simulink library "MicDiagBtc"  (R2022b)
settings: Solver=VariableStepAuto  StartTime=0.0  StopTime=10.0  RelTol=1e-3
libraries: RTC x2, FeaturePath x1, HandyTextFile x1, simulink x1
settings Model: Creator=yp1048186  LastModifiedBy=kl13806
settings SolverCC: AlgebraicLoopSolver=TrustRegion
settings DebuggingCC: UnconnectedInputMsg=warning  UnconnectedOutputMsg=warning  UnconnectedLineMsg=warning  SFMachineParentedDataDiag=warning
settings ModelReferenceCC: EnableRefExpFcnMdlSchedulingChecks=on
settings RTWCC: DLArmComputeVersion=19.05

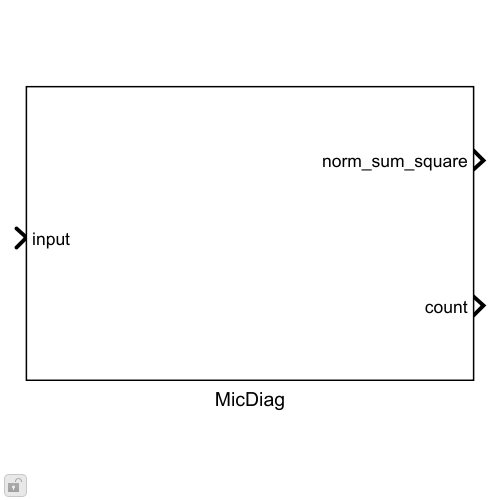
[thumbnail: Simulink's stored preview of the top-level diagram]
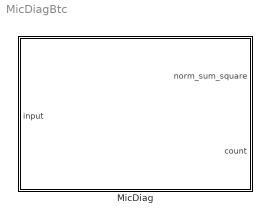
== system MicDiagBtc ==
  MicDiag : Subsystem  mask(Blocklib MicDiag){Config=[], FeatureName=MicDiag}
      mask prompts: Config "MicDiagConfig"; FeatureName "Feature path name:"
      mask help: MicDiag accumulates the sum of squares for multiple channels individually
      mask init:
      | blkh=gcbh;
      | Config=BTConfig.Assert(blkh,Config);
      | 
      | Config.Validate();
      | BTConfig.InitSetFeatureIfPresent(blkh,'FeatureName');
      mask Callback Config: BTConfig.CallbackHideIfPresent(gcbh,{'FeatureName'});
      mask TypeOptions FeatureName: FeaturePath/FeatureName

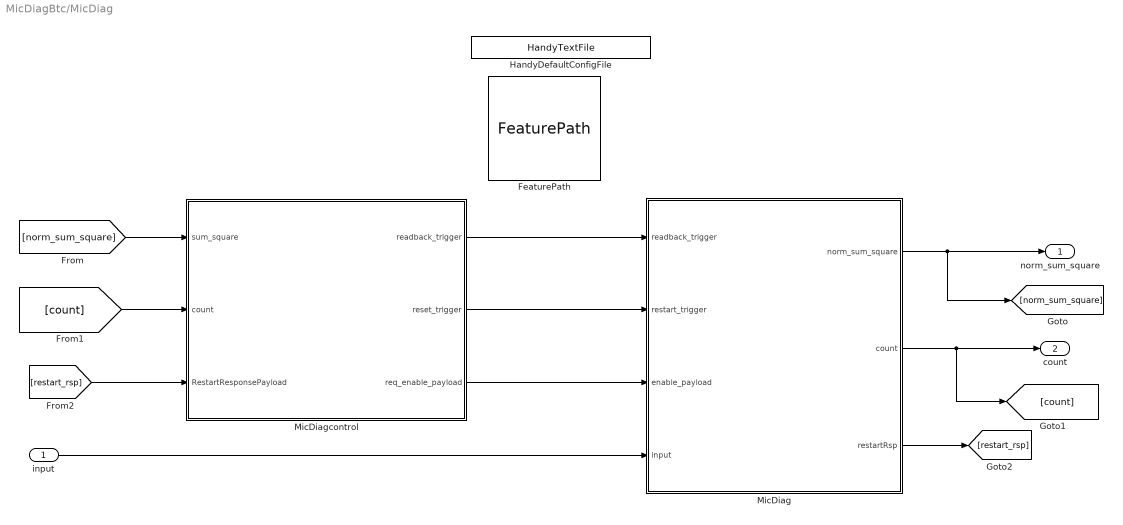
== system MicDiagBtc/MicDiag ==
  input : Inport
  FeaturePath : FeaturePath/FeaturePath  FeatureName=MicDiag  IsGroup=off  GroupNumber=-1  IsModule=off  TriggerInit=[485 19 600 126]
  HandyDefaultConfigFile : HandyTextFile/HandyTextFile  TemplateSource=Config  FileSuffix=Init  OpenDialogOnLoad=off  UseThisBlockName=off  TheDefaultText=|  ShowInLibBrowser=on
      | % $(FILENAME) Setup model parameters for each "Init" callback (e.g. update diagram)
      | sample_rate_in_hertz = 44100;
      | frame_size = 32;
      | sysin_channel_count = 2;
  MicDiag : Subsystem
  MicDiagcontrol : Subsystem
  norm_sum_square : Outport
  count : Outport  Port=2
  wires:
  [restart_rsp] -> MicDiagcontrol/3(RestartResponsePayload)
  MicDiagcontrol/3(req_enable_payload) -> MicDiag/3(enable_payload)
  MicDiag/3(restartRsp) -> [restart_rsp]
  [norm_sum_square] -> MicDiagcontrol/1(sum_square)
  MicDiagcontrol/1(readback_trigger) -> MicDiag/1(readback_trigger)
  MicDiagcontrol/2(reset_trigger) -> MicDiag/2(restart_trigger)
  MicDiag/1(norm_sum_square) -> norm_sum_square/1, [norm_sum_square]
  input/1 -> MicDiag/4(input)
  MicDiag/2(count) -> count/1, [count]
  [count] -> MicDiagcontrol/2(count)

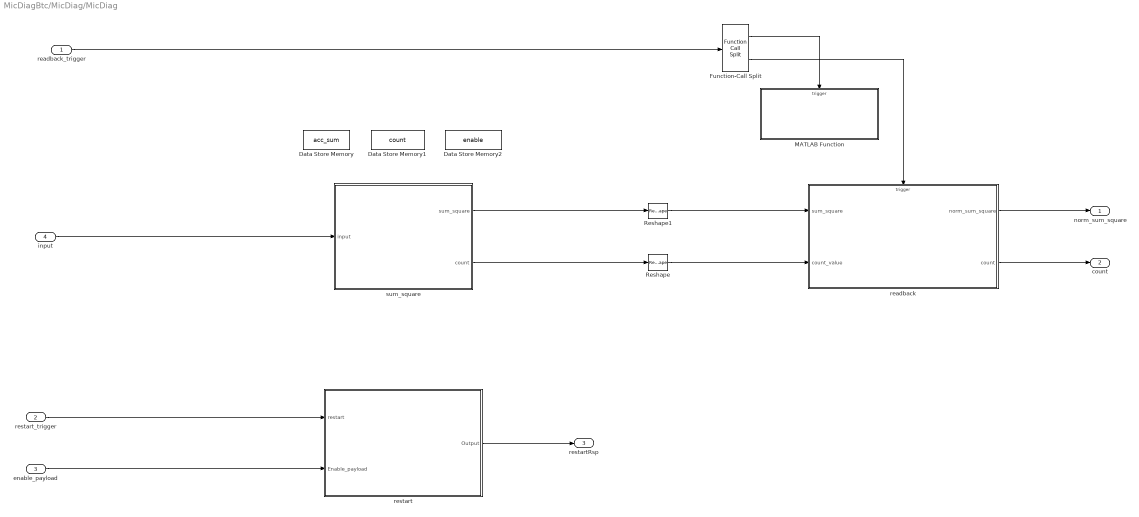
== system MicDiagBtc/MicDiag/MicDiag ==
  readback_trigger : Inport
  restart_trigger : Inport  Port=2
  enable_payload : Inport  Port=3
  input : Inport  Port=4
  Data Store Memory : DataStoreMemory  DataStoreName=acc_sum  InitialValue=zeros(Config.NumMicIn,1)  ShowAdditionalParam=off  OutDataTypeStr=single
  Data Store Memory1 : DataStoreMemory  DataStoreName=count  InitialValue=zeros(Config.NumMicIn,1)  ShowAdditionalParam=off  OutDataTypeStr=int32
  Data Store Memory2 : DataStoreMemory  DataStoreName=enable  InitialValue=zeros(Config.NumMicIn,1)  ShowAdditionalParam=off  OutDataTypeStr=int32
  Function-Call Split : FunctionCallSplit  IconShape=distinctive  NumOutputPorts=2
  MATLAB Function : MATLAB Function  TreatAsAtomicUnit=on
  Reshape : Reshape  OutputDimensionality=Row vector (2-D)
  Reshape1 : Reshape  OutputDimensionality=Row vector (2-D)
  readback : Subsystem  TreatAsAtomicUnit=on
  restart : Subsystem
  sum_square : Subsystem
  norm_sum_square : Outport
  count : Outport  Port=2
  restartRsp : Outport  Port=3
  wires:
  restart/1(Output) -> restartRsp/1
  Function-Call Split/1 -> MATLAB Function/Trigger
  Function-Call Split/2 -> readback/Trigger
  readback_trigger/1 -> Function-Call Split/1
  readback/1(norm_sum_square) -> norm_sum_square/1
  readback/2(count) -> count/1
  input/1 -> sum_square/1(input)
  restart_trigger/1 -> restart/1(restart)
  enable_payload/1 -> restart/2(Enable_payload)
  sum_square/1(sum_square) -> Reshape1/1
  sum_square/2(count) -> Reshape/1
  Reshape1/1 -> readback/1(sum_square)
  Reshape/1 -> readback/2(count_value)

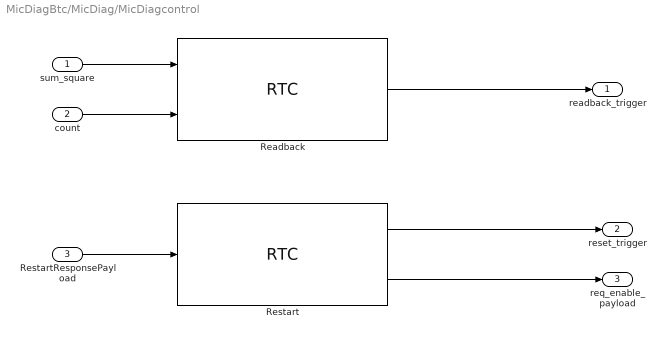
== system MicDiagBtc/MicDiag/MicDiagcontrol ==
  sum_square : Inport
  count : Inport  Port=2
  RestartResponsePayload : Inport  Port=3
  Readback : RTC/RTC  REQ_Priority=RTC_Mask.NormalPriority  RequestAtInit=off  EnableRequest=on  REQElemType1=uint32  REQElemWidth1=1  REQElemInitial1=[]  REQElemType2=uint32  REQElemWidth2=1  REQElemInitial2=[]  REQElemType3=uint32  REQElemWidth3=1  REQElemInitial3=[]  REQElemType4=uint32  REQElemWidth4=1  REQElemInitial4=[]  REQElemType5=uint32  REQElemWidth5=1  REQElemInitial5=[]  REQElemType6=uint32  REQElemWidth6=1  REQElemInitial6=[]  REQElemType7=uint32  REQElemWidth7=1  REQElemInitial7=[]  REQElemType8=uint32  REQElemWidth8=1  REQElemInitial8=[]  REQElemType9=uint32  REQElemWidth9=1  REQElemInitial9=[]  REQElemType10=uint32  REQElemWidth10=1  REQElemInitial10=[]  EnableResponse=on  EnableRSP_StatusIn=off  RSPElemName1=sum_square  RSPElemType1=uint32  RSPElemWidth1=Config.NumMicIn  RSPElemName2=count  RSPElemType2=uint32  RSPElemWidth2=Config.NumMicIn  RSPElemType3=uint32  RSPElemWidth3=1  RSPElemType4=uint32  RSPElemWidth4=1  RSPElemType5=uint32  RSPElemWidth5=1  RSPElemType6=uint32  RSPElemWidth6=1  RSPElemType7=uint32  RSPElemWidth7=1  RSPElemType8=uint32  RSPElemWidth8=1  RSPElemType9=uint32  RSPElemWidth9=1  RSPElemType10=uint32  RSPElemWidth10=1  EnableNotification=off  EnableNTF_PrepTrig=off  NTFElemType1=uint32  NTFElemWidth1=1  NTFElemType2=uint32  NTFElemWidth2=1  NTFElemType3=uint32  NTFElemWidth3=1  NTFElemType4=uint32  NTFElemWidth4=1  NTFElemType5=uint32  NTFElemWidth5=1  NTFElemType6=uint32  NTFElemWidth6=1  NTFElemType7=uint32  NTFElemWidth7=1  NTFElemType8=uint32  NTFElemWidth8=1  NTFElemType9=uint32  NTFElemWidth9=1  NTFElemType10=uint32  NTFElemWidth10=1  MaskMessageName=Readback
  Restart : RTC/RTC  REQ_Priority=RTC_Mask.NormalPriority  RequestAtInit=off  EnableRequest=on  REQElemName1=enable  REQElemType1=int32  REQElemWidth1=Config.NumMicIn  REQElemInitial1=[]  REQElemType2=uint32  REQElemWidth2=1  REQElemInitial2=[]  REQElemType3=uint32  REQElemWidth3=1  REQElemInitial3=[]  REQElemType4=uint32  REQElemWidth4=1  REQElemInitial4=[]  REQElemType5=uint32  REQElemWidth5=1  REQElemInitial5=[]  REQElemType6=uint32  REQElemWidth6=1  REQElemInitial6=[]  REQElemType7=uint32  REQElemWidth7=1  REQElemInitial7=[]  REQElemType8=uint32  REQElemWidth8=1  REQElemInitial8=[]  REQElemType9=uint32  REQElemWidth9=1  REQElemInitial9=[]  REQElemType10=uint32  REQElemWidth10=1  REQElemInitial10=[]  EnableResponse=on  EnableRSP_StatusIn=off  RSPElemName1=RestartResponsePayload  RSPElemType1=int32  RSPElemWidth1=1  RSPElemType2=uint32  RSPElemWidth2=1  RSPElemType3=uint32  RSPElemWidth3=1  RSPElemType4=uint32  RSPElemWidth4=1  RSPElemType5=uint32  RSPElemWidth5=1  RSPElemType6=uint32  RSPElemWidth6=1  RSPElemType7=uint32  RSPElemWidth7=1  RSPElemType8=uint32  RSPElemWidth8=1  RSPElemType9=uint32  RSPElemWidth9=1  RSPElemType10=uint32  RSPElemWidth10=1  EnableNotification=off  EnableNTF_PrepTrig=off  NTFElemType1=uint32  NTFElemWidth1=1  NTFElemType2=uint32  NTFElemWidth2=1  NTFElemType3=uint32  NTFElemWidth3=1  NTFElemType4=uint32  NTFElemWidth4=1  NTFElemType5=uint32  NTFElemWidth5=1  NTFElemType6=uint32  NTFElemWidth6=1  NTFElemType7=uint32  NTFElemWidth7=1  NTFElemType8=uint32  NTFElemWidth8=1  NTFElemType9=uint32  NTFElemWidth9=1  NTFElemType10=uint32  NTFElemWidth10=1  MaskMessageName=Restart
  readback_trigger : Outport
  reset_trigger : Outport  Port=2
  req_enable_payload : Outport  Port=3
  wires:
  RestartResponsePayload/1 -> Restart/1
  sum_square/1 -> Readback/1
  Restart/1 -> reset_trigger/1
  Readback/1 -> readback_trigger/1
  Restart/2 -> req_enable_payload/1
  count/1 -> Readback/2

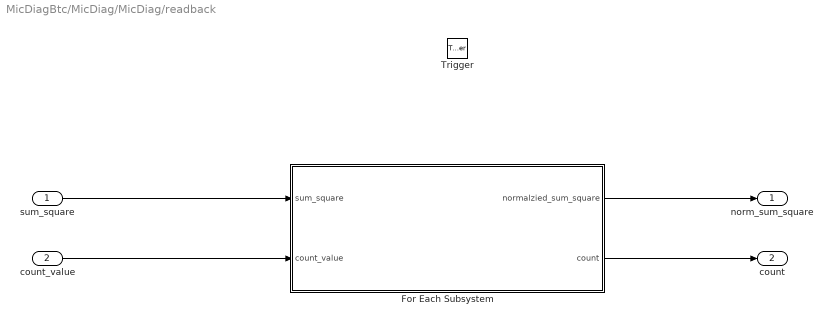
== system MicDiagBtc/MicDiag/MicDiag/readback ==
  sum_square : Inport
  count_value : Inport  Port=2
  Trigger : TriggerPort  TriggerType=function-call  VariantControl=Variant
  For Each Subsystem : Subsystem  TreatAsAtomicUnit=on
  norm_sum_square : Outport  InitialOutput=zeros(Config.NumMicIn,1)
  count : Outport  Port=2  InitialOutput=zeros(Config.NumMicIn,1)
  wires:
  sum_square/1 -> For Each Subsystem/1(sum_square)
  count_value/1 -> For Each Subsystem/2(count_value)
  For Each Subsystem/2(count) -> count/1
  For Each Subsystem/1(normalzied_sum_square) -> norm_sum_square/1

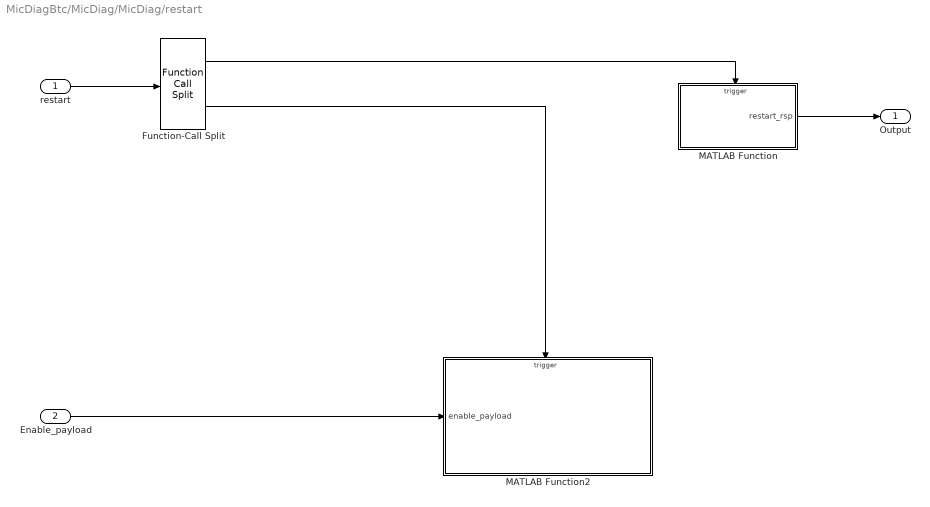
== system MicDiagBtc/MicDiag/MicDiag/restart ==
  restart : Inport
  Enable_payload : Inport  Port=2
  Function-Call Split : FunctionCallSplit  IconShape=distinctive  NumOutputPorts=2  OutputPortLayout=default
  MATLAB Function : MATLAB Function  TreatAsAtomicUnit=on
  MATLAB Function2 : MATLAB Function  TreatAsAtomicUnit=on
  Output : Outport
  wires:
  MATLAB Function/1(restart_rsp) -> Output/1
  Function-Call Split/1 -> MATLAB Function/Trigger
  restart/1 -> Function-Call Split/1
  Function-Call Split/2 -> MATLAB Function2/Trigger
  Enable_payload/1 -> MATLAB Function2/1(enable_payload)

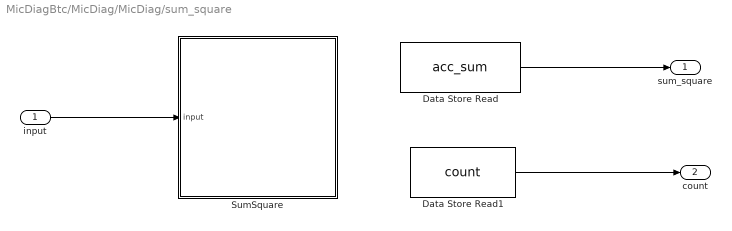
== system MicDiagBtc/MicDiag/MicDiag/sum_square ==
  input : Inport
  Data Store Read : DataStoreRead  DataStoreName=acc_sum  IndexOptions=Index vector (dialog)  Indices=1  OutputSizes=1
  Data Store Read1 : DataStoreRead  DataStoreName=count  IndexOptions=Index vector (dialog)  Indices=1  OutputSizes=1
  SumSquare : MATLAB Function  TreatAsAtomicUnit=on
  sum_square : Outport
  count : Outport  Port=2
  wires:
  input/1 -> SumSquare/1(input)
  Data Store Read/1 -> sum_square/1
  Data Store Read1/1 -> count/1

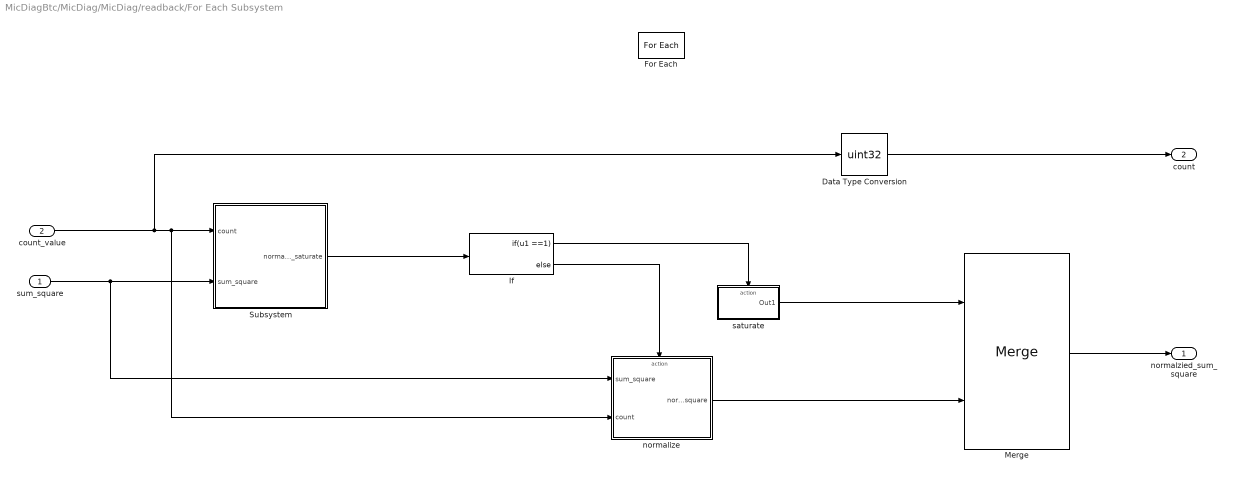
== system MicDiagBtc/MicDiag/MicDiag/readback/For Each Subsystem ==
  sum_square : Inport  Partition=on  PartitionDimension=2  PartitionWidth=1  PartitionOffset=0
  count_value : Inport  Port=2  Partition=on  PartitionDimension=2  PartitionWidth=1  PartitionOffset=0
  Data Type Conversion : DataTypeConversion  OutDataTypeStr=uint32  RndMeth=Nearest  SaturateOnIntegerOverflow=off
  For Each : ForEach  DisableCoverage=on
  If : If  IfExpression=u1 ==1
  Merge : Merge
  Subsystem : Subsystem
  normalize : Subsystem  TreatAsAtomicUnit=on
  saturate : Subsystem  TreatAsAtomicUnit=on
  normalzied_sum_square : Outport  OutputWhenDisabled=reset  InitialOutput=[0]  ConcatenationDimension=1  VectorParamsAs1DForOutWhenUnconnected=off
  count : Outport  Port=2  OutputWhenDisabled=reset  InitialOutput=[0]  ConcatenationDimension=1  VectorParamsAs1DForOutWhenUnconnected=off
  wires:
  Subsystem/1(normalize_saturate) -> If/1
  If/1 -> saturate/Action
  count_value/1 -> Data Type Conversion/1, Subsystem/1(count), normalize/2(count)
  normalize/1(normalize_sum_square) -> Merge/2
  saturate/1(Out1) -> Merge/1
  sum_square/1 -> Subsystem/2(sum_square), normalize/1(sum_square)
  Merge/1 -> normalzied_sum_square/1
  Data Type Conversion/1 -> count/1
  If/2 -> normalize/Action

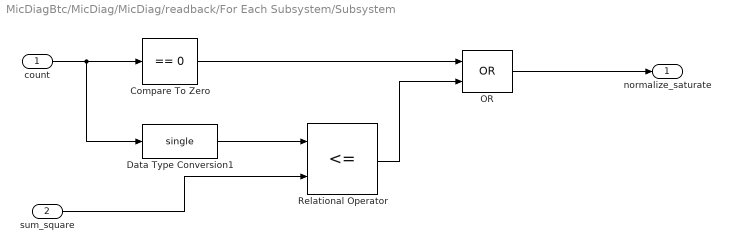
== system MicDiagBtc/MicDiag/MicDiag/readback/For Each Subsystem/Subsystem ==
  count : Inport
  sum_square : Inport  Port=2
  Compare To Zero : simulink/Logic and Bit Operations/Compare To Zero  relop===  OutDataTypeStr=boolean
  Data Type Conversion1 : DataTypeConversion  OutDataTypeStr=single  SaturateOnIntegerOverflow=off  RndMeth=Floor
  OR : Logic  Operator=OR  IconShape=distinctive  AllPortsSameDT=off  OutDataTypeStr=boolean
  Relational Operator : RelationalOperator  Operator=<=  OutDataTypeStr=boolean  RndMeth=Simplest  InputSameDT=off
  normalize_saturate : Outport
  wires:
  Data Type Conversion1/1 -> Relational Operator/1
  Compare To Zero/1 -> OR/1
  OR/1 -> normalize_saturate/1
  sum_square/1 -> Relational Operator/2
  count/1 -> Compare To Zero/1, Data Type Conversion1/1
  Relational Operator/1 -> OR/2

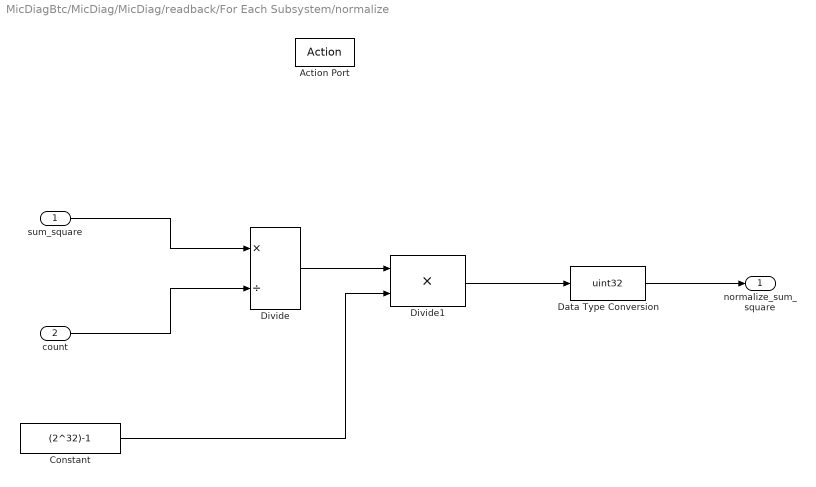
== system MicDiagBtc/MicDiag/MicDiag/readback/For Each Subsystem/normalize ==
  sum_square : Inport
  count : Inport  Port=2
  Action Port : ActionPort
  Constant : Constant  Value=(2^32)-1  OutDataTypeStr=single
  Data Type Conversion : DataTypeConversion  OutDataTypeStr=uint32  SaturateOnIntegerOverflow=off  RndMeth=Floor
  Divide : Product  Inputs=*/
  Divide1 : Product
  normalize_sum_square : Outport
  wires:
  Data Type Conversion/1 -> normalize_sum_square/1
  Divide1/1 -> Data Type Conversion/1
  Constant/1 -> Divide1/2
  Divide/1 -> Divide1/1
  count/1 -> Divide/2
  sum_square/1 -> Divide/1

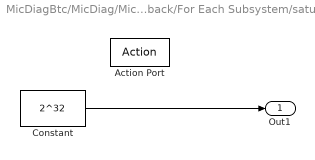
== system MicDiagBtc/MicDiag/MicDiag/readback/For Each Subsystem/saturate ==
  Action Port : ActionPort
  Constant : Constant  Value=2^32  OutDataTypeStr=uint32
  Out1 : Outport
  wires:
  Constant/1 -> Out1/1

== matlab function MicDiagBtc/MicDiag/MicDiag/MATLAB Function ==
  data: enable data_store_memory
  events: trigger input FUNCTION_CALL_EVENT
function ReadbackDisableAccumulation
    %#codegen
    % datastore memory to control the audio processing logic:
    global enable;
    % find the size of the enable 
    numIn = length(enable);
    % When Readback is requested,accumulation of sum of sqaure shall freeze
    enable = int32(zeros(numIn,1));
end

== matlab function MicDiagBtc/MicDiag/MicDiag/sum_square/SumSquare ==
  data: input input single size=[framesize numMicIn]; acc_sum data_store_memory; count data_store_memory; enable data_store_memory
function sumsquare(input)
    %#codegen
    % datastore memory to control the audio processing logic:
    global acc_sum;
    global count;
    global enable;
    % number of mic
    numMicIn = size(input,2);
    % frame size
    framesize = size(input,1);
    % Compute sum_of_squares and count
    % if corresponding mic is enabled(which is a RTC message) 
    for MicIn = 1:numMicIn
        if(enable(MicIn) == 1)
            acc_sum(MicIn) = acc_sum(MicIn)+ sum(input(:,MicIn).^2);
            count(MicIn) = count(MicIn)+ framesize;
        end
    end

== matlab function MicDiagBtc/MicDiag/MicDiag/restart/MATLAB Function ==
  data: restart_rsp output int32 size=1
  events: trigger input FUNCTION_CALL_EVENT
function restart_rsp = GenRestartRsp 
% Return the restart reponse as 1
   restart_rsp = int32(1);

== matlab function MicDiagBtc/MicDiag/MicDiag/restart/MATLAB Function2 ==
  data: count data_store_memory; enable data_store_memory; acc_sum data_store_memory; enable_payload input int32 size=numMicIn
  events: trigger input FUNCTION_CALL_EVENT
function restart(enable_payload)
    %#codegen
    % datastore memory to control the audio processing logic:
    global acc_sum;
    global count;
    global enable;
    
    %Fetch the num of the microphone 
    numMicIn  = length(acc_sum);
    
    % freeze the accumulation by clearing enable
    enable = int32(zeros(numMicIn,1));
    % clear accumulator
    acc_sum(1:numMicIn)= single(zeros(numMicIn,1));
    % clear count
    count(1:numMicIn)  = int32(zeros(numMicIn,1));
    
    %unfreeze the accumulation by setting the enable to the paylaod value
    for idx = 1:numMicIn
        if(enable_payload(idx)==1)
            enable(idx) = enable_payload(idx);
        end
    end
